simulink library "LumArduinoBlockset_Due"  (R2016b)
settings: Solver=VariableStepAuto  StartTime=0.0  StopTime=10.0  RelTol=1e-3  EnableMultiTasking=on
values from neighbouring files (symbols this model uses):
  T = varargin{2}    [IncrementalRotaryEncoder.m]
undefined symbols (not defined in the file or in its folder): a
libraries: arduinolib x8, UWArduinoBlockset_Due x8
settings Model: Creator=Christopher  LastModifiedBy=chris
settings DataIOCC: LimitDataPoints=on
settings OptimizationCC: LifeSpan=inf
settings DebuggingCC: AllowSymbolicDim=off  SFUnexpectedBacktrackingDiag=warning  SFNoUnconditionalDefaultTransitionDiag=warning  SFExecutionAtInitializationDiag=none
settings ModelReferenceCC: PropagateSignalLabelsOutOfModel=off
settings GRTTargetCC: TargetLangStandard=C89/C90 (ANSI)
settings ConfigComp: CovMetricSettings=dw  CovHtmlReporting=on  CovSaveCumulativeToWorkspaceVar=on  CovSaveSingleToWorkspaceVar=on  CovExternalEMLEnable=off

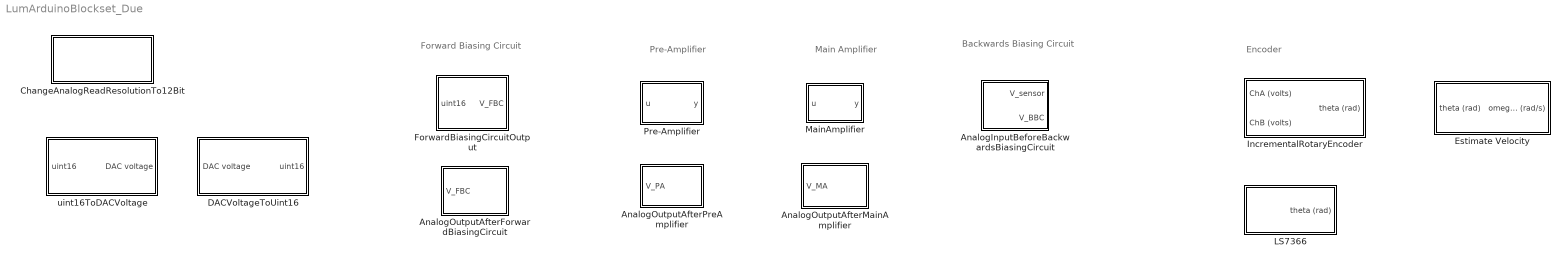
== system LumArduinoBlockset_Due ==
  note: Backwards Biasing Circuit
  note: Main Amplifier
  note: Encoder
  note: Pre-Amplifier
  note: Forward Biasing Circuit
  AnalogInputBeforeBackwardsBiasingCircuit : Subsystem  mask{P1=0.33113, P2=1.64, pinNumber=7, T=T}
      mask prompts: pinNumber "Analog Input Pin Number"; T "Sample Time (seconds)"
      mask help:
      | This operates similar to the 'Analog Input' block in the sense that it reads voltages that are input to the Arduino system.  This block outputs the voltage that was input to the BBC (typically the voltage output by the sensor).
      |
      | This assumes the following:
      | -The backwards biasing circuit is connected to the pin specified
      | -The input/ouput relationship of the BBC is V_BBC = P1*V_sensor + P2
      | -The analog input resolution has been set to 12-bits (see 'ChangeAnalogReadResolutionTo12Bit' block)
      |
      | INPUT:	None
      |
      | OUTPUT:	V_sensor:	voltage input to the BBC (typically from a sensor), should not exceeld [-5,5] volts (volts)
      | 	V_BBC:	voltage output by the BBC (volts)
      |
      | Created by Christopher Lum
      | lum@uw.edu
  AnalogOutputAfterForwardBiasingCircuit : Subsystem
      mask help:
      | This operates similar to the 'Analog Output' block in the sense that it allows the user to specify voltages that will be output by the Forward Biasing Circuit (FBC).
      |
      | Note that V_FBC should be in the range of [-1.1,1.1] volts.  Values are saturated to this range.
      |
      | This assumes the following:
      | -The input to the FBC is connected to DAC1 of the Arduino
      |
      | INPUT:  V_FBC:  desired voltage to be output by the FBC (volts)
      |
      | Created by Christopher Lum
      | lum@uw.edu
  AnalogOutputAfterMainAmplifier : Subsystem  mask{K_preamp=6, K_kepco=-3.6}
      mask prompts: K_preamp "Pre-amplifier gain"; K_kepco "Main amplifier gain (typically negative)"
      mask help:
      | This operates similar to the 'Analog Output' block in the sense that it allows the user to specify voltages that will be ouput by the main amplifier (the Kepco).
      |
      |
      | This assumes the following:
      | -The main amplifier is connected in series after the pre-amplifier.
      | -All pre-requisites/assumptions specified by the AnalogOutputAfterPreAmplifier block are satisfied
      |
      | INPUT:  V_MA:  desired voltage to be output by the main amplifier (volts)
      |
      | Created by Christopher Lum
      | lum@uw.edu
  AnalogOutputAfterPreAmplifier : Subsystem  mask{K_preamp=6}
      mask prompts: K_preamp "Pre-amplifier gain"
      mask help:
      | This operates similar to the 'Analog Output' block in the sense that it allows the user to specify voltages that will be output by pre-amplifier.
      |
      | This assumes the following:
      | -The pre-amplifier is connected in series after the Forward Biasing Circuit.
      | -All pre-requisites/assumptions specified by the AnalogOutputAfterForwardBiasingCircuit block are satisfied
      |
      | INPUT:  V_PA:  desired voltage to be output by the pre-amplifier (volts)
      |
      | Created by Christopher Lum
      | lum@uw.edu
  ChangeAnalogReadResolutionTo12Bit : Subsystem
      mask help:
      | When this block is included in the model, it will change the resolution of the analog in pins to 12-bits.
      |
      | Note that upon building this block, several files named 'setAnalogReadResolution' will be created in the working directory.
      |
      | Christopher Lum
      | lum@uw.edu
      |
      | Original block by Robert Freiholtz (http://robertfreiholtz.se/simulink-arduino-due-change-10-bits-to-12-bits-analogread)
  DACVoltageToUint16 : Subsystem
      mask help:
      | Computes the value needed to be input to the DAC0 or DAC1 in order to obtained the desired voltage.
      |
      | The desired voltage value is saturated to [0.55,2.75] volts.
      |
      | INPUT:  DAC voltage: voltage desired to be output by DAC0 or DAC1 (volts)
      |
      | OUTPUT: uint16: uint16 value that needs to be sent to the 'Analog Output' block (DAC0 or DAC1) (uint16)
      |
      | Created by Christopher Lum
      | lum@uw.edu
  Estimate Velocity : Subsystem  mask{a=a}
      mask prompts: a "Pseudo-derivative frequency (rad/s)"
      mask help:
      | Estimate the velocity using a pseudo-derivative.
      |
      | INPUT:	theta:	motor angle (rad)
      |
      | OUTPUT:	omega:	motor velocity (rad/s)
      |
      | Created by Christopher Lum
      | lum@uw.edu
  ForwardBiasingCircuitOutput : Subsystem
      mask help:
      | This block predicts the voltage that will be output after the forward biasing circuit (FBC).
      |
      | This assumes the following:
      | -DAC0 from the Arduino is connected to the V_in of the FBC
      | -DAC1 from the Arduino is connected to the V_offset of the FBC and outputs 1.65 volts (offset voltage)
      |
      | INPUT:  -uint16: uint16 value sent to DAC0
      |
      | OUTPUT: -V_FBC:  voltage output from the FBC (volts)
      |
      | Created by Christopher Lum
      | lum@uw.edu
  IncrementalRotaryEncoder : Subsystem  mask{N=500}
      mask prompts: N "N (number lines per revolution of encoder)"
      mask help:
      | This reads an incremental, quadrature encoder and converts to angle.
      |
      | INPUT:  ChA:    channel A voltage (volts)
      |         ChB:    channel B voltage (volts)
      |
      | OUTPUT: theta:  angle of the encoder (rad)
      |
      | Created by Christopher Lum
      | lum@uw.edu
  LS7366 : Subsystem  mask{N=500, T=T}
      mask prompts: N "Number lines per revolution of encoder"; T "Sample time (seconds)"
      mask help:
      | Interfaces with the LS7366 chip to read the encoder counts.
      |
      | This block places the LS7366 in 4x quadrature, 4-byte mode.
      |
      | Note that for the Due, the slave select (SS) from the LS7366 must be connected to D4, D10, or D52.
      |
      | This assumes the following:
      | LS7366 slave select (SS) is connected to Due pin D52.
      |
      | INPUT:	none
      |
      | OUTPUT:	angle of the encoder, theta (rad)
      |
      | Created by Christopher Lum
      | lum@uw.edu
  MainAmplifier : Subsystem  mask{K_kepco=-3.6}
      mask prompts: K_kepco "Amplifier gain (typically negative)"
      mask help:
      | Models the main power amplifier (the Kepco).
      |
      | INPUT:  u: input voltage to the amplifier (volts)
      |
      | OUTPUT: y: output voltage from the amplifier (volts)
      |
      | Created by Christopher Lum
      | lum@uw.edu
  Pre-Amplifier : Subsystem  mask{K_preamp=6}
      mask prompts: K_preamp "Amplifier gain"
      mask help:
      | Models the pre-amplifier.
      |
      | INPUT:  u: input voltage to the pre-amplifier
      |
      | OUTPUT: y: output voltage from the pre-amplifier
      |
      | Created by Christopher Lum
      | lum@uw.edu
  uint16ToDACVoltage : Subsystem
      mask help:
      | Computes the value that the DAC0 or DAC1 will output when the specified input is given to the 'Analog Output' block.
      |
      | This accounts for the overflow/wrap-around of the 16 bit value to a 12-bit range.
      |
      | INPUT:  uint16: input uint16 sent to the 'Analog Output' block (DAC0 or DAC1) (uint16)
      |
      | OUTPUT: DAC voltage: voltage output by DAC0 or DAC1 (volts)
      |
      | Created by Christopher Lum
      | lum@uw.edu

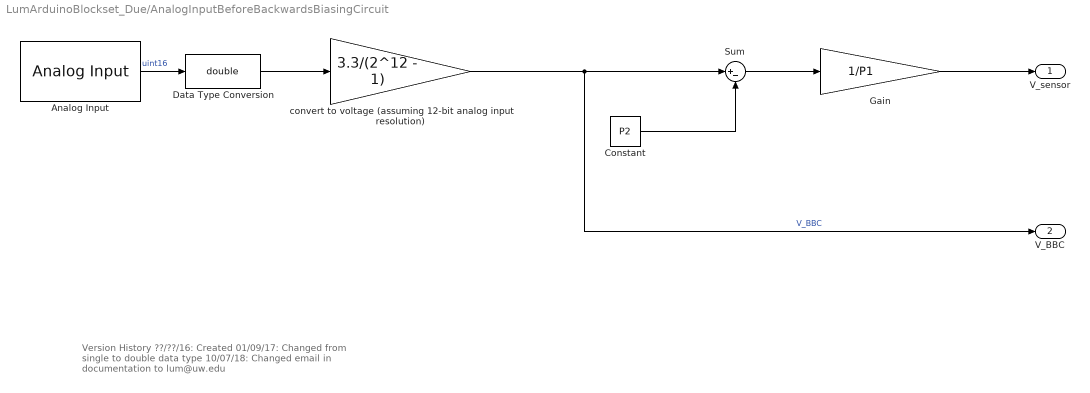
== system LumArduinoBlockset_Due/AnalogInputBeforeBackwardsBiasingCircuit ==
  note: Version History
      | ??/??/16: Created
      | 01/09/17: Changed from single to double data type
      | 10/07/18:  Changed email in documentation to lum@uw.edu
  Analog Input : arduinolib/Analog Input  pinNumber=pinNumber  sampleTime=T  blockPlatform=arduino
  Constant : Constant  Value=P2
  Data Type Conversion : DataTypeConversion  OutDataTypeStr=double
  Gain : Gain  Gain=1/P1
  Sum : Sum  Inputs=|+-
  convert to voltage (assuming 12-bit analog input resolution) : Gain  Gain=3.3/(2^12 - 1)
  V_sensor : Outport
  V_BBC : Outport  Port=2
  wires:
  Constant/1 -> Sum/2
  Sum/1 -> Gain/1
  Gain/1 -> V_sensor/1
  Analog Input/1 -> Data Type Conversion/1  "uint16"
  Data Type Conversion/1 -> convert to voltage (assuming 12-bit analog input resolution)/1
  convert to voltage (assuming 12-bit analog input resolution)/1 -> V_BBC/1, Sum/1  "V_BBC"

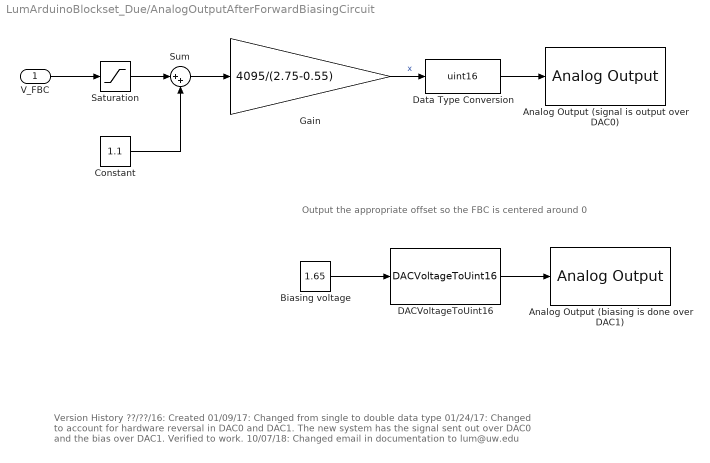
== system LumArduinoBlockset_Due/AnalogOutputAfterForwardBiasingCircuit ==
  note: Version History
      | ??/??/16: Created
      | 01/09/17: Changed from single to double data type
      | 01/24/17: Changed to account for hardware reversal in DAC0 and DAC1.  The new system has the signal sent out over DAC0 and the bias over DAC1.  Verified to work.
      | 10/07/18:  Changed email in documentation to lum@uw.edu
  note: Output the appropriate offset so the FBC is centered around 0
  V_FBC : Inport
  Analog Output (biasing is done over DAC1) : arduinolib/Analog Output  DACpin=DAC1  blockPlatform=arduino
  Analog Output (signal is output over DAC0) : arduinolib/Analog Output  DACpin=DAC0  blockPlatform=arduino
  Biasing voltage : Constant  Value=1.65
  Constant : Constant  Value=1.1
  DACVoltageToUint16 : UWArduinoBlockset_Due/DACVoltageToUint16
  Data Type Conversion : DataTypeConversion  OutDataTypeStr=uint16
  Gain : Gain  Gain=4095/(2.75-0.55)
  Saturation : Saturate  UpperLimit=1.1  LowerLimit=-1.1
  Sum : Sum  Inputs=|++
  wires:
  V_FBC/1 -> Saturation/1
  Constant/1 -> Sum/2
  Sum/1 -> Gain/1
  Saturation/1 -> Sum/1
  Gain/1 -> Data Type Conversion/1  "x"
  Data Type Conversion/1 -> Analog Output (signal is output over DAC0)/1
  DACVoltageToUint16/1 -> Analog Output (biasing is done over DAC1)/1
  Biasing voltage/1 -> DACVoltageToUint16/1

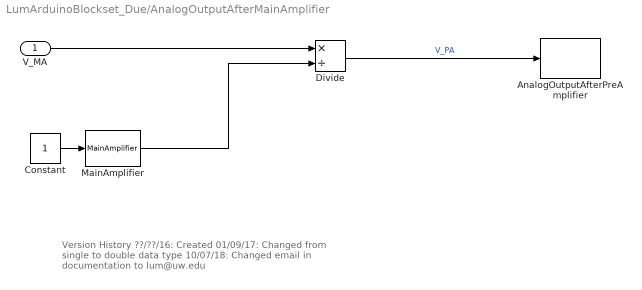
== system LumArduinoBlockset_Due/AnalogOutputAfterMainAmplifier ==
  note: Version History
      | ??/??/16:  Created
      | 01/09/17:  Changed from single to double data type
      | 10/07/18:  Changed email in documentation to lum@uw.edu
  V_MA : Inport
  AnalogOutputAfterPreAmplifier : UWArduinoBlockset_Due/AnalogOutputAfterPreAmplifier  K_preamp=K_preamp
  Constant : Constant
  Divide : Product  Inputs=*/
  MainAmplifier : UWArduinoBlockset_Due/MainAmplifier  K_kepco=K_kepco
  wires:
  V_MA/1 -> Divide/1
  Constant/1 -> MainAmplifier/1
  MainAmplifier/1 -> Divide/2
  Divide/1 -> AnalogOutputAfterPreAmplifier/1  "V_PA"

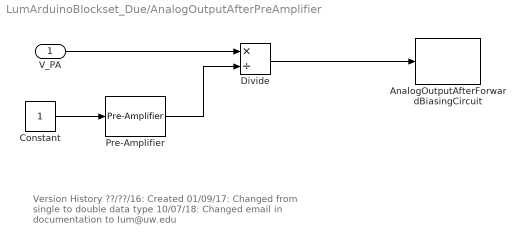
== system LumArduinoBlockset_Due/AnalogOutputAfterPreAmplifier ==
  note: Version History
      | ??/??/16: Created
      | 01/09/17: Changed from single to double data type
      | 10/07/18:  Changed email in documentation to lum@uw.edu
  V_PA : Inport
  AnalogOutputAfterForwardBiasingCircuit : UWArduinoBlockset_Due/AnalogOutputAfterForwardBiasingCircuit
  Constant : Constant
  Divide : Product  Inputs=*/
  Pre-Amplifier : UWArduinoBlockset_Due/Pre-Amplifier  K_preamp=K_preamp
  wires:
  V_PA/1 -> Divide/1
  Constant/1 -> Pre-Amplifier/1
  Pre-Amplifier/1 -> Divide/2
  Divide/1 -> AnalogOutputAfterForwardBiasingCircuit/1

== system LumArduinoBlockset_Due/ChangeAnalogReadResolutionTo12Bit ==
  note: Version History:
      | 12/18/14: Initial version by Robert Freiholtz
      | 11/15/16: Created block
      | 12/28/16: Allowed block to modify its contents thereby allowing automatic generation of necessary files.
      | 01/16/17: Moved version history documentation underneath the mask.
      | 10/07/18: Changed email in documentation to lum@uw.edu
  Constant : Constant  Value=0
  trigger to setAnalogReadResolution to 12 bits : S-Function  InitFcn=try, set_param(gcb,'FunctionName','setAnalogReadResolution'), end  FunctionName=setAnalogReadResolution  SFunctionModules=setAnalogReadResolution_wrapper  SFunctionDeploymentMode=off  EnableBusSupport=off  mask(S-Function Builder){}
      mask help: Simulink:masks:SFunctionBuilder_MD
      mask init:
      | val = [[.9  0.75 0.75 1 1 .9 .9 1]',[1 1 0.75 0.75 .9 .9 1 .9]'];try , sys = get_param(gcb,'SfunBuilderFcnName');if isempty(sys), sys = get_param(gcb,'FunctionName'); end,catch, sys = get_param(gcb,'FunctionName'); end
      settings: CopyFcn=set_param(gcbh,'LinkStatus','none')  PreSaveFcn=try, set_param(gcb,'FunctionName','setAnalogReadResolution'), end  OpenFcn=sfunctionwizard(gcbh)
      mask Display: plot(val(:,1),val(:,2)),disp(sys), port_label('input',1,'trigger')
  wires:
  Constant/1 -> trigger to setAnalogReadResolution to 12 bits/1

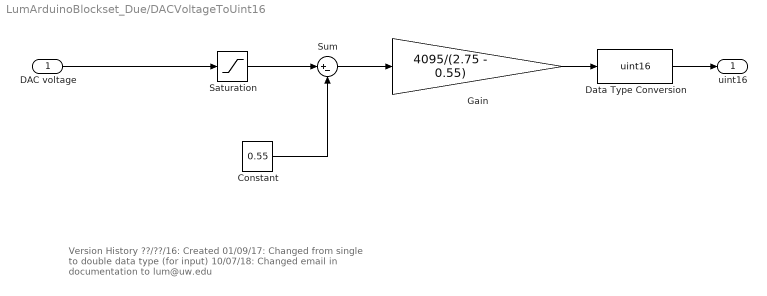
== system LumArduinoBlockset_Due/DACVoltageToUint16 ==
  note: Version History
      | ??/??/16: Created
      | 01/09/17: Changed from single to double data type (for input)
      | 10/07/18:  Changed email in documentation to lum@uw.edu
  DAC voltage : Inport
  Constant : Constant  Value=0.55
  Data Type Conversion : DataTypeConversion  OutDataTypeStr=uint16
  Gain : Gain  Gain=4095/(2.75 - 0.55)
  Saturation : Saturate  UpperLimit=2.75  LowerLimit=.55
  Sum : Sum  Inputs=|+-
  uint16 : Outport
  wires:
  Saturation/1 -> Sum/1
  Constant/1 -> Sum/2
  DAC voltage/1 -> Saturation/1
  Sum/1 -> Gain/1
  Gain/1 -> Data Type Conversion/1
  Data Type Conversion/1 -> uint16/1

== system LumArduinoBlockset_Due/Estimate Velocity ==
  note: Version History:
      | ??/??/??:  Created
      | 10/07/18:  Changed email in documentation to lum@uw.edu
  theta (rad) : Inport
  Transfer Fcn : TransferFcn  Numerator=[a^2 0]  Denominator=[1 2*a a^2]
  omega (rad/s) : Outport
  wires:
  theta (rad)/1 -> Transfer Fcn/1
  Transfer Fcn/1 -> omega (rad/s)/1

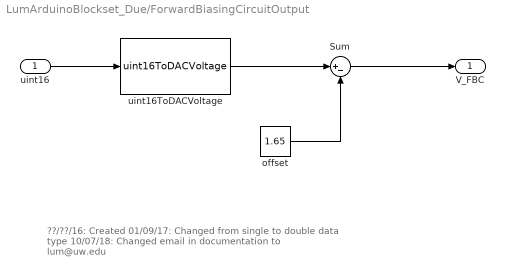
== system LumArduinoBlockset_Due/ForwardBiasingCircuitOutput ==
  note: ??/??/16: Created
      | 01/09/17: Changed from single to double data type
      | 10/07/18:  Changed email in documentation to lum@uw.edu
  uint16 : Inport
  Sum : Sum  Inputs=|+-
  offset : Constant  Value=1.65
  uint16ToDACVoltage : UWArduinoBlockset_Due/uint16ToDACVoltage
  V_FBC : Outport
  wires:
  uint16/1 -> uint16ToDACVoltage/1
  uint16ToDACVoltage/1 -> Sum/1
  offset/1 -> Sum/2
  Sum/1 -> V_FBC/1

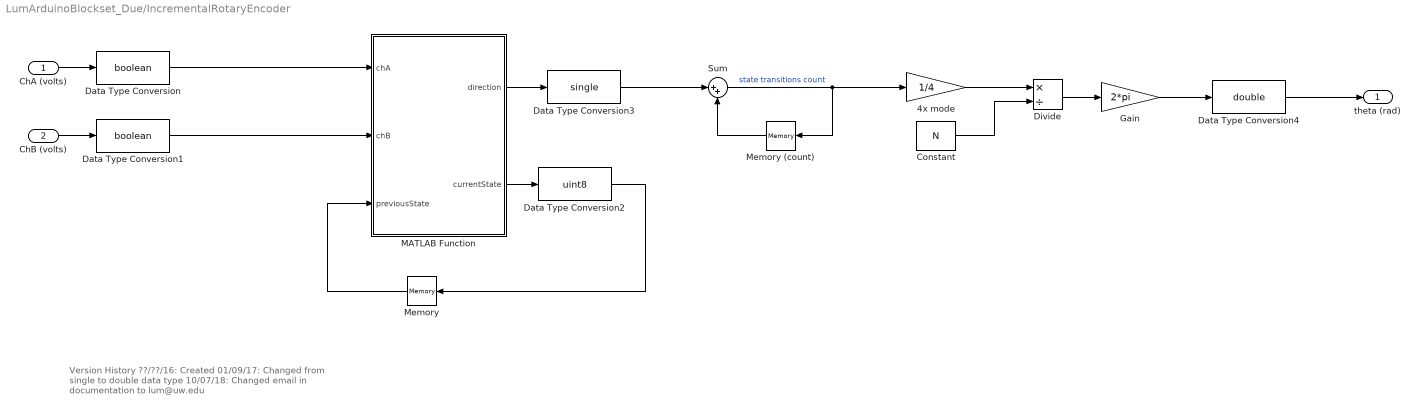
== system LumArduinoBlockset_Due/IncrementalRotaryEncoder ==
  note: Version History
      | ??/??/16:  Created
      | 01/09/17:  Changed from single to double data type
      | 10/07/18:  Changed email in documentation to lum@uw.edu
  ChA (volts) : Inport
  ChB (volts) : Inport  Port=2
  4x mode : Gain  Gain=1/4
  Constant : Constant  Value=N  OutDataTypeStr=single
  Data Type Conversion : DataTypeConversion  OutDataTypeStr=boolean
  Data Type Conversion1 : DataTypeConversion  OutDataTypeStr=boolean
  Data Type Conversion2 : DataTypeConversion  OutDataTypeStr=uint8
  Data Type Conversion3 : DataTypeConversion  OutDataTypeStr=single
  Data Type Conversion4 : DataTypeConversion  OutDataTypeStr=double
  Divide : Product  Inputs=*/
  Gain : Gain  Gain=2*pi
  MATLAB Function : MATLAB Function  TreatAsAtomicUnit=on
  Memory : Memory  X0=1
  Memory (count) : Memory
  Sum : Sum  Inputs=|++
  theta (rad) : Outport
  wires:
  ChB (volts)/1 -> Data Type Conversion1/1
  ChA (volts)/1 -> Data Type Conversion/1
  MATLAB Function/1(direction) -> Data Type Conversion3/1
  MATLAB Function/2(currentState) -> Data Type Conversion2/1
  Memory/1 -> MATLAB Function/3(previousState)
  Data Type Conversion/1 -> MATLAB Function/1(chA)
  Data Type Conversion1/1 -> MATLAB Function/2(chB)
  Data Type Conversion2/1 -> Memory/1
  Data Type Conversion3/1 -> Sum/1
  Memory (count)/1 -> Sum/2
  Sum/1 -> Memory (count)/1, 4x mode/1  "state transitions count"
  Divide/1 -> Gain/1
  Constant/1 -> Divide/2
  Gain/1 -> Data Type Conversion4/1
  4x mode/1 -> Divide/1
  Data Type Conversion4/1 -> theta (rad)/1

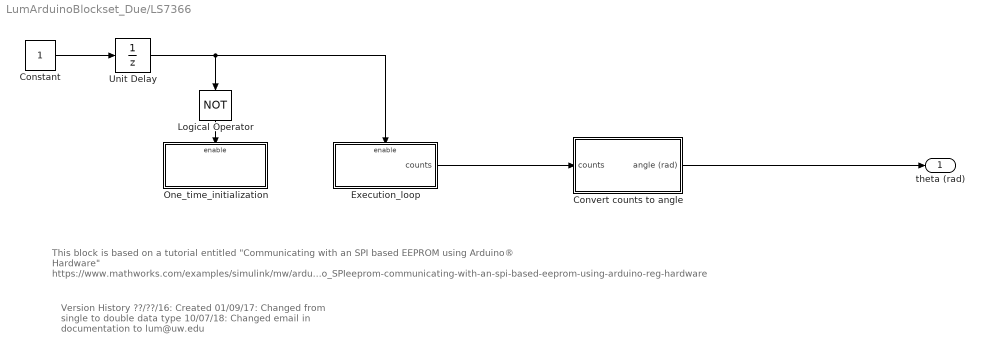
== system LumArduinoBlockset_Due/LS7366 ==
  note: Version History
      | ??/??/16:  Created
      | 01/09/17:  Changed from single to double data type
      | 10/07/18:  Changed email in documentation to lum@uw.edu
  note: This block is based on a tutorial entitled "Communicating with an SPI based EEPROM using Arduino® Hardware"
      | https://www.mathworks.com/examples/simulink/mw/arduino_product-arduino_SPIeeprom-communicating-with-an-spi-based-eeprom-using-arduino-reg-hardware
  Constant : Constant  OutDataTypeStr=boolean  SampleTime=T
  Convert counts to angle : Subsystem
  Execution_loop : Subsystem  TreatAsAtomicUnit=on
  Logical Operator : Logic  Operator=NOT  AllPortsSameDT=off  OutDataTypeStr=boolean
  One_time_initialization : Subsystem  TreatAsAtomicUnit=on
  Unit Delay : UnitDelay  SampleTime=-1
  theta (rad) : Outport
  wires:
  Constant/1 -> Unit Delay/1
  Unit Delay/1 -> Execution_loop/Enable, Logical Operator/1
  Logical Operator/1 -> One_time_initialization/Enable
  Execution_loop/1(counts) -> Convert counts to angle/1(counts)
  Convert counts to angle/1(angle (rad)) -> theta (rad)/1

== system LumArduinoBlockset_Due/MainAmplifier ==
  note: Version History:
      | ??/??/16:  Created
      | 10/07/18:  Changed email in documentation to lum@uw.edu
  u : Inport
  Gain : Gain  Gain=K_kepco
  y : Outport
  wires:
  u/1 -> Gain/1
  Gain/1 -> y/1

== system LumArduinoBlockset_Due/Pre-Amplifier ==
  note: Version History:
      | ??/??/16: Created
      | 10/07/18:  Changed email in documentation to lum@uw.edu
  u : Inport
  Gain : Gain  Gain=K_preamp
  y : Outport
  wires:
  u/1 -> Gain/1
  Gain/1 -> y/1

== system LumArduinoBlockset_Due/uint16ToDACVoltage ==
  note: Version History
      | ??/??/16: Created
      | 01/09/17: Changed output to double instead of single data type
      | 10/07/18:  Changed email in documentation to lum@uw.edu
  uint16 : Inport
  MATLAB Function : MATLAB Function  TreatAsAtomicUnit=on
  DAC voltage : Outport
  wires:
  uint16/1 -> MATLAB Function/1(u)
  MATLAB Function/1(y) -> DAC voltage/1

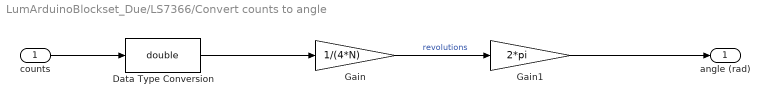
== system LumArduinoBlockset_Due/LS7366/Convert counts to angle ==
  counts : Inport
  Data Type Conversion : DataTypeConversion  OutDataTypeStr=double
  Gain : Gain  Gain=1/(4*N)
  Gain1 : Gain  Gain=2*pi
  angle (rad) : Outport
  wires:
  Data Type Conversion/1 -> Gain/1
  Gain/1 -> Gain1/1  "revolutions"
  counts/1 -> Data Type Conversion/1
  Gain1/1 -> angle (rad)/1

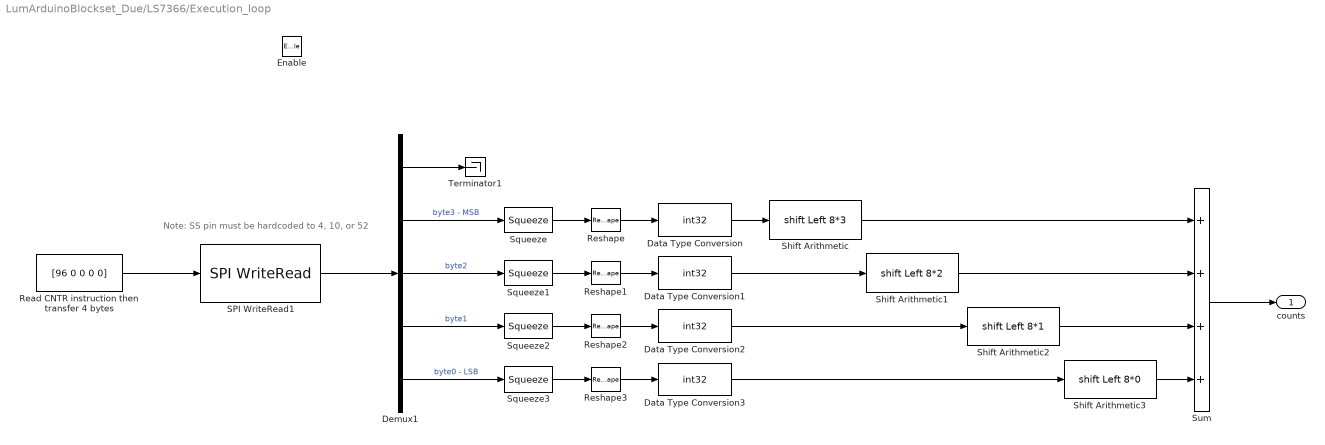
== system LumArduinoBlockset_Due/LS7366/Execution_loop ==
  note: Note: SS pin must be hardcoded to 4, 10, or 52
  Enable : EnablePort  StatesWhenEnabling=reset
  Data Type Conversion{,1..3} (4 alike) : DataTypeConversion  OutDataTypeStr=int32
  Demux1 : Demux  Outputs=5
  Read CNTR instruction then transfer 4 bytes : Constant  Value=[96 0 0 0 0]  OutDataTypeStr=uint8  SampleTime=T
  Reshape{,1..3} (4 alike) : Reshape
  SPI WriteRead1 : arduinolib/SPI WriteRead  slaveSelectPin_=52  blockPlatform=arduino
  Shift Arithmetic : ArithShift  BitShiftNumber=8*3  BitShiftDirection=Left
  Shift Arithmetic1 : ArithShift  BitShiftNumber=8*2  BitShiftDirection=Left
  Shift Arithmetic2 : ArithShift  BitShiftNumber=8*1  BitShiftDirection=Left
  Shift Arithmetic3 : ArithShift  BitShiftNumber=8*0  BitShiftDirection=Left
  Squeeze{,1..3} (4 alike) : Squeeze
  Sum : Sum  Inputs=++++
  Terminator1 : Terminator
  counts : Outport  InitialOutput=0
  wires:
  SPI WriteRead1/1 -> Demux1/1
  Demux1/1 -> Terminator1/1
  Demux1/2 -> Squeeze/1  "byte3 - MSB"
  Demux1/3 -> Squeeze1/1  "byte2"
  Demux1/4 -> Squeeze2/1  "byte1"
  Demux1/5 -> Squeeze3/1  "byte0 - LSB"
  Shift Arithmetic/1 -> Sum/1
  Shift Arithmetic1/1 -> Sum/2
  Shift Arithmetic2/1 -> Sum/3
  Shift Arithmetic3/1 -> Sum/4
  Data Type Conversion/1 -> Shift Arithmetic/1
  Data Type Conversion1/1 -> Shift Arithmetic1/1
  Data Type Conversion2/1 -> Shift Arithmetic2/1
  Data Type Conversion3/1 -> Shift Arithmetic3/1
  Read CNTR instruction then transfer 4 bytes/1 -> SPI WriteRead1/1
  Squeeze/1 -> Reshape/1
  Reshape/1 -> Data Type Conversion/1
  Reshape1/1 -> Data Type Conversion1/1
  Squeeze1/1 -> Reshape1/1
  Reshape2/1 -> Data Type Conversion2/1
  Squeeze2/1 -> Reshape2/1
  Reshape3/1 -> Data Type Conversion3/1
  Squeeze3/1 -> Reshape3/1
  Sum/1 -> counts/1

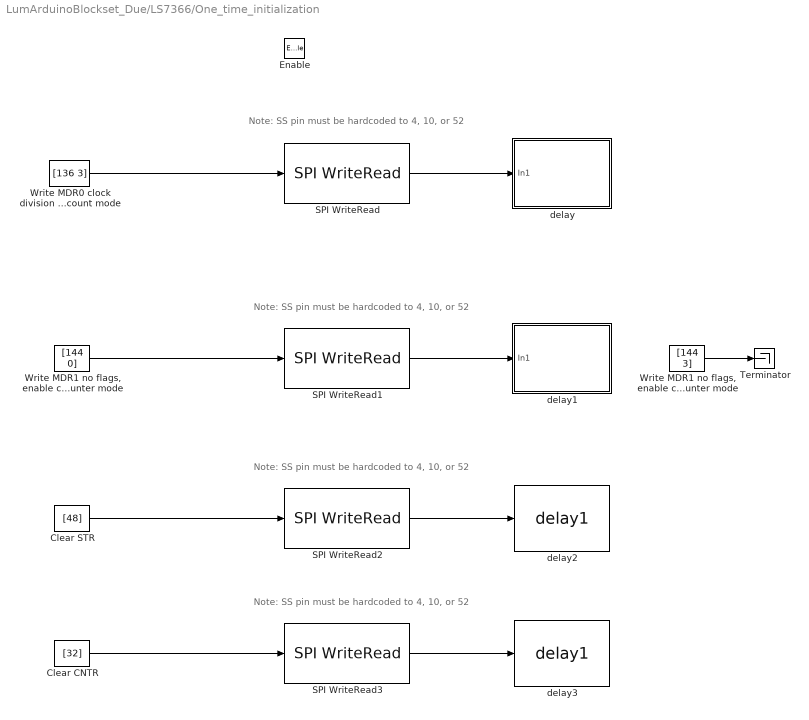
== system LumArduinoBlockset_Due/LS7366/One_time_initialization ==
  note: Note: SS pin must be hardcoded to 4, 10, or 52
  note: Note: SS pin must be hardcoded to 4, 10, or 52
  note: Note: SS pin must be hardcoded to 4, 10, or 52
  note: Note: SS pin must be hardcoded to 4, 10, or 52
  Enable : EnablePort  StatesWhenEnabling=reset
  Clear CNTR : Constant  Value=[32]  OutDataTypeStr=uint8  SampleTime=T
  Clear STR : Constant  Value=[48]  OutDataTypeStr=uint8  SampleTime=T
  SPI WriteRead{,1..3} (4 alike) : arduinolib/SPI WriteRead  slaveSelectPin_=52  blockPlatform=arduino
  Terminator : Terminator
  "Write MDR0 clock division factor = 1, negative index input, disable index, free-running count mode, 4x quadrature count mode" : Constant  Value=[136 3]  OutDataTypeStr=uint8  SampleTime=T
  "Write MDR1 no flags, enable counting, 1-byte counter mode " : Constant  Value=[144 3]  OutDataTypeStr=uint8  SampleTime=T
  "Write MDR1 no flags, enable counting, 4-byte counter mode" : Constant  Value=[144 0]  OutDataTypeStr=uint8  SampleTime=T
  delay : Subsystem  Priority=1
      settings: AttributesFormatString=Priority=%<Priority>
  delay1 : Subsystem
  delay2 : UWArduinoBlockset_Due/LS7366/One_time_initialization/delay1
  delay3 : UWArduinoBlockset_Due/LS7366/One_time_initialization/delay1
  wires:
  "Write MDR0 clock division factor = 1, negative index input, disable index, free-running count mode, 4x quadrature count mode"/1 -> SPI WriteRead/1
  SPI WriteRead/1 -> delay/1(In1)
  SPI WriteRead1/1 -> delay1/1(In1)
  "Write MDR1 no flags, enable counting, 4-byte counter mode"/1 -> SPI WriteRead1/1
  "Write MDR1 no flags, enable counting, 1-byte counter mode "/1 -> Terminator/1
  SPI WriteRead2/1 -> delay2/1
  Clear STR/1 -> SPI WriteRead2/1
  SPI WriteRead3/1 -> delay3/1
  Clear CNTR/1 -> SPI WriteRead3/1

== system LumArduinoBlockset_Due/LS7366/One_time_initialization/delay ==
  In1 : Inport
  Subsystem : Subsystem
  Terminator : Terminator
  wires:
  Subsystem/1(Out1) -> Terminator/1
  In1/1 -> Subsystem/1(In1)

== system LumArduinoBlockset_Due/LS7366/One_time_initialization/delay1 ==
  In1 : Inport
  Subsystem : Subsystem
  Terminator : Terminator
  wires:
  In1/1 -> Subsystem/1(In1)
  Subsystem/1(Out1) -> Terminator/1

== system LumArduinoBlockset_Due/LS7366/One_time_initialization/delay/Subsystem ==
  In1 : Inport
  For Iterator : ForIterator  IterationLimit=10000  ShowIterationPort=off  IndexMode=Zero-based
  Gain : Gain  OutDataTypeStr=Inherit: Same as input  ParamDataTypeStr=Inherit: Same as input
  Out1 : Outport
  wires:
  In1/1 -> Gain/1
  Gain/1 -> Out1/1

== system LumArduinoBlockset_Due/LS7366/One_time_initialization/delay1/Subsystem ==
  In1 : Inport
  For Iterator : ForIterator  IterationLimit=10000  ShowIterationPort=off  IndexMode=Zero-based
  Gain : Gain  OutDataTypeStr=Inherit: Same as input  ParamDataTypeStr=Inherit: Same as input
  Out1 : Outport
  wires:
  Gain/1 -> Out1/1
  In1/1 -> Gain/1

== matlab function LumArduinoBlockset_Due/IncrementalRotaryEncoder/MATLAB Function ==
  data: chA input; direction output; chB input; currentState output; previousState input
function [direction, currentState] = fcn(chA, chB, previousState)
%#codegen

%Determines if the encoder moved CCW, CW, or is inconsistent
%
%INPUT: chA:            channel A state (boolean)
%       chB:            channel B state (boolean)
%       previousState:  previous state of encoder (1, 2, 3, or 4) (uint8)
%
%OUPUT: direction:      1 = CCW, -1 = CW, 0 = no rotation or inconsistent (int8)
%       currentState:   current state of encoder (1, 2, 3, or 4) (uint8)

%Determine current state of the encoder
if(~chA && ~chB)
    currentState = 1;
    
elseif(~chA && chB)
    currentState = 2;
    
elseif(chA && chB)
    currentState = 3;
    
elseif(chA && ~chB)
    currentState = 4;
    
else
    error('Unknown currentState of encoder!')
    
end
    
%Compare with previous state to determine which way the encoder turned
if(previousState==1)
    if(currentState==1)
        %No rotation
        direction = 0;
        
    elseif(currentState==2)
        %CCW rotation
        direction = 1;
        
    elseif(currentState==4)
        %CW rotation
        direction = -1;
        
    else
        %inconsistent state transition, do nothing
        direction = 0;
    end
    
elseif(previousState==2)
    if(currentState==2)
        %No rotation
        direction = 0;
        
    elseif(currentState==3)
        %CCW rotation
        direction = 1;
        
    elseif(currentState==1)
        %CW rotation
        direction = -1;
        
    else
        %inconsistent state transition, do nothing
        direction = 0;
    end
    
elseif(previousState==3)
    if(currentState==3)
        %No rotation
        direction = 0;
        
    elseif(currentState==4)
        %CCW rotation
        direction = 1;
        
    elseif(currentState==2)
        %CW rotation
        direction = -1;
        
    else
        %inconsistent state transition, do nothing
        direction = 0;
    end
    
elseif(previousState==4)
    if(currentState==4)
        %No rotation
        direction = 0;
        
    elseif(currentState==1)
        %CCW rotation
        direction = 1;
        
    elseif(currentState==3)
        %CW rotation
        direction = -1;
        
    else
        %inconsistent state transition, do nothing
        direction = 0;
    end
    
else
    error('previousState is not known!')
end

== matlab function LumArduinoBlockset_Due/uint16ToDACVoltage/MATLAB Function ==
  data: u input; y output
function y = fcn(u)
%#codegen

%Wrap the input to the range [0, 4095]
maxVal = 2^12 - 1;
uTilde = mod(double(u), maxVal + 1);

%Map the int to a voltage
yMin = 0.55;
yMax = 2.75;

rise = yMax - yMin;
run = maxVal;
m = rise/run;

y = m*uTilde + yMin;
